simulink model "Roadsense_SemanticPerception"  (R2025b)
settings: Solver=FixedStepDiscrete  StartTime=0.0  StopTime=0.1  FixedStep=RsTsBase  RelTol=1e-3
undefined symbols (not defined in the file or in its folder): RsCameraImageHeight, RsCameraImageWidth, RsTsSemanticInference
settings Model: DataDictionary=Roadsense_Data.sldd  Creator=ragur  LastModifiedBy=ragur

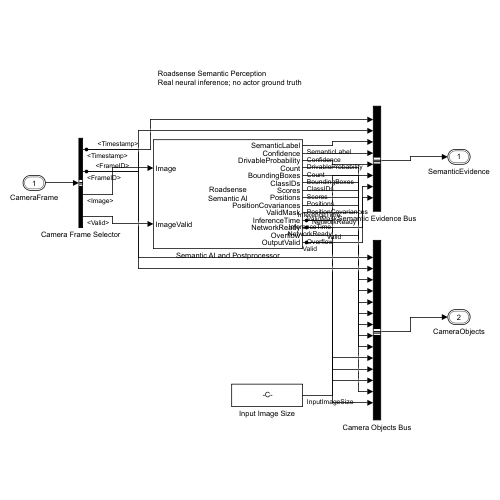
[thumbnail: Simulink's stored preview of the top-level diagram]
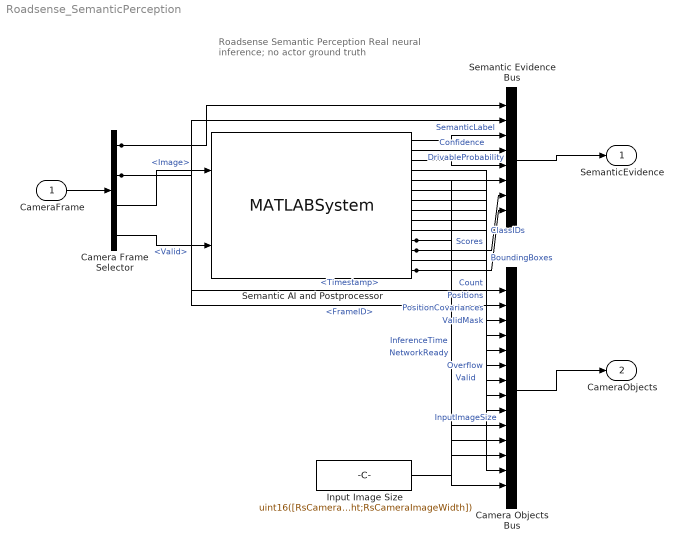
== system Roadsense_SemanticPerception ==
  note: Roadsense Semantic Perception
      | Real neural inference; no actor ground truth
  CameraFrame : Inport  OutDataTypeStr=Bus: RsCameraFrameBus  PortDimensions=1  SampleTime=RsTsSemanticInference
  Camera Frame Selector : BusSelector  OutputSignals=Timestamp,FrameID,Image,Valid
  Camera Objects Bus : BusCreator  Inputs=14  OutDataTypeStr=Bus: RsCameraObjectListBus
  Input Image Size : Constant  Value=uint16([RsCameraImageHeight;RsCameraImageWidth])  OutDataTypeStr=uint16
  Semantic AI and Postprocessor : MATLABSystem  System=RoadsenseSemanticPerceptionSystem  ExecutionEnvironment=cpu  InferenceMode=syntheticColor  MinimumConfidence=single(0.449999988079071)  MinimumBlobArea=uint32(60)  FocalLength=single([400;400])  PrincipalPoint=single([319.5;239.5])  CameraHeight=single(1.39999997615814)  CameraPitchDown=single(0.0872664600610733)  MaximumGroundRange=single(80)  SimulateUsing=Interpreted execution
      mask Type: RoadsenseSemanticPerceptionSystem
  Semantic Evidence Bus : BusCreator  Inputs=8  OutDataTypeStr=Bus: RsImageSemanticBus
  SemanticEvidence : Outport  OutDataTypeStr=Bus: RsImageSemanticBus
  CameraObjects : Outport  Port=2  OutDataTypeStr=Bus: RsCameraObjectListBus
  wires:
  CameraFrame/1 -> Camera Frame Selector/1
  Camera Frame Selector/3 -> Semantic AI and Postprocessor/1  "<Image>"
  Camera Frame Selector/4 -> Semantic AI and Postprocessor/2  "<Valid>"
  Camera Frame Selector/1 -> Semantic Evidence Bus/1, Camera Objects Bus/1  "<Timestamp>"
  Camera Frame Selector/2 -> Semantic Evidence Bus/2, Camera Objects Bus/2  "<FrameID>"
  Semantic AI and Postprocessor/1 -> Semantic Evidence Bus/3  "SemanticLabel"
  Semantic AI and Postprocessor/2 -> Semantic Evidence Bus/4  "Confidence"
  Semantic AI and Postprocessor/3 -> Semantic Evidence Bus/5  "DrivableProbability"
  Semantic AI and Postprocessor/11 -> Semantic Evidence Bus/6, Camera Objects Bus/11  "InferenceTime"
  Semantic AI and Postprocessor/12 -> Semantic Evidence Bus/7, Camera Objects Bus/12  "NetworkReady"
  Semantic AI and Postprocessor/14 -> Semantic Evidence Bus/8, Camera Objects Bus/14  "Valid"
  Semantic AI and Postprocessor/4 -> Camera Objects Bus/3  "Count"
  Semantic AI and Postprocessor/5 -> Camera Objects Bus/4  "BoundingBoxes"
  Semantic AI and Postprocessor/6 -> Camera Objects Bus/5  "ClassIDs"
  Semantic AI and Postprocessor/7 -> Camera Objects Bus/6  "Scores"
  Semantic AI and Postprocessor/8 -> Camera Objects Bus/7  "Positions"
  Semantic AI and Postprocessor/9 -> Camera Objects Bus/8  "PositionCovariances"
  Semantic AI and Postprocessor/10 -> Camera Objects Bus/9  "ValidMask"
  Input Image Size/1 -> Camera Objects Bus/10  "InputImageSize"
  Semantic AI and Postprocessor/13 -> Camera Objects Bus/13  "Overflow"
  Semantic Evidence Bus/1 -> SemanticEvidence/1
  Camera Objects Bus/1 -> CameraObjects/1
